simulink model "model_zad3"  (R2023a)
settings: Solver=ode45  StartTime=0.0  StopTime=600  RelTol=1e-3  EnableMultiTasking=on
values from neighbouring files (symbols this model uses):
  theta = [Gd.den{1}(2:3) Gd.num{1}(2:3)]'    [inicijalizacija.m]
  theta2 = [Gd2.den{1}(2:3) Gd2.num{1}(2:3)]'    [inicijalizacija.m]
  Ts = dt    [inicijalizacija.m]
libraries: simulink x2
settings Model: Creator=starcic  LastModifiedBy=Enio
settings SolverCC: AlgebraicLoopSolver=TrustRegion
settings DataIOCC: LimitDataPoints=on  SaveFormat=Array  ReturnWorkspaceOutputs=off
settings OptimizationCC: LifeSpan=inf
settings DebuggingCC: UnderspecifiedInitializationDetection=Classic  MergeDetectMultiDrivingBlocksExec=none  SolverPrmCheckMsg=warning  FcnCallInpInsideContextMsg=warning  UnconnectedInputMsg=warning  UnconnectedOutputMsg=warning  UnconnectedLineMsg=warning  StateNameClashWarn=warning  SFUnexpectedBacktrackingDiag=warning  SFNoUnconditionalDefaultTransitionDiag=warning  SFExecutionAtInitializationDiag=none  ArithmeticOperatorsInVariantConditions=warning
settings HardwareCC: ProdBitPerPointer=32  ProdBitPerSizeT=32  ProdBitPerPtrDiffT=32  ProdLargestAtomicFloat=None  ProdIntDivRoundTo=Undefined  ProdEndianess=Unspecified  ProdWordSize=32  ProdHWDeviceType=32-bit Generic
settings ModelReferenceCC: PropagateSignalLabelsOutOfModel=off
settings SFSimCC: SimUseLocalCustomCode=off  CustomCodeUndefinedFunction=UseInterfaceOnly
settings RTWCC: RTWUseLocalCustomCode=off
settings CodeAppCC: StateflowObjectComments=on
settings GRTTargetCC: TargetLangStandard=C89/C90 (ANSI)  CombineOutputUpdateFcns=off  GRTInterface=on
settings ConfigComp: CovMetricSettings=dw  CovSaveCumulativeToWorkspaceVar=on  CovSaveSingleToWorkspaceVar=on  CovExternalEMLEnable=off

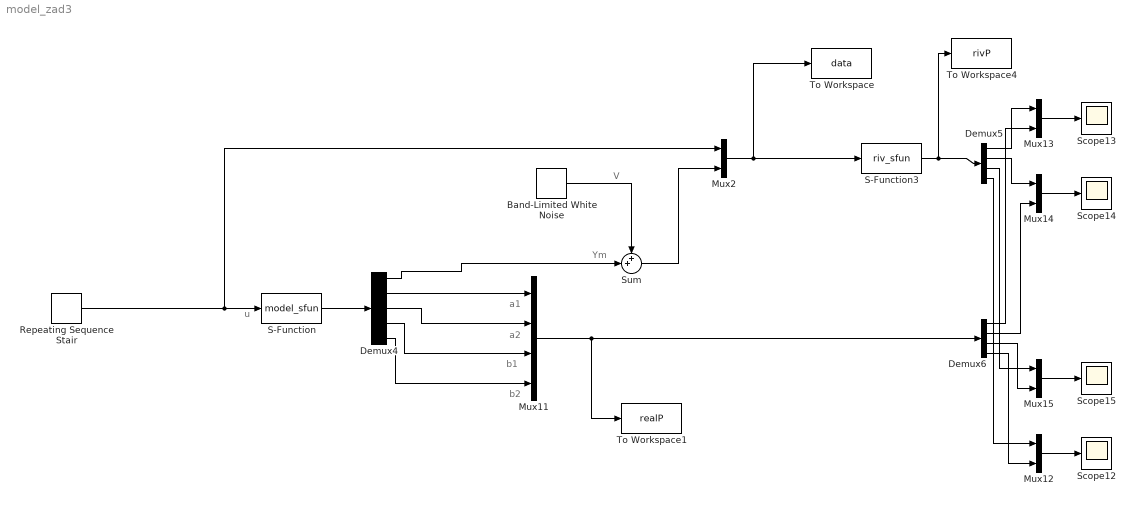
== system model_zad3 ==
  note: V
  note: u
  note: Ym
  note: b2
  note: b1
  note: a2
  note: a1
  Band-Limited White Noise : simulink/Sources/Band-Limited White Noise  Cov=[0.0000001]  Ts=Ts  seed=145656456
  Demux4 : Demux  Outputs=5
  Demux5 : Demux
  Demux6 : Demux
  Mux11 : Mux
  Mux{2,12..15} (5 alike) : Mux  Inputs=2
  Repeating Sequence Stair : simulink/Sources/Repeating Sequence Stair  OutValues=ui  tsamp=Ts  OutMin=[]  OutMax=[]  OutDataTypeStr=double  OutputDataTypeScalingMode=double  OutDataType=fixdt(0,8)  ConRadixGroup=Best Precision: Vector-wise  OutScaling=2^-12
  S-Function : S-Function  FunctionName=model_sfun  Parameters=theta,theta2  SFunctionDeploymentMode=off  EnableBusSupport=off
  S-Function3 : S-Function  FunctionName=riv_sfun  Parameters=Ts  SFunctionDeploymentMode=off  EnableBusSupport=off
  Scope{12..15} (4 alike) : Scope
  Sum : Sum  Inputs=++|
  To Workspace : ToWorkspace  VariableName=data  SaveFormat=Structure With Time  SampleTime=Ts
  To Workspace1 : ToWorkspace  VariableName=realP  SaveFormat=Structure With Time  SampleTime=Ts
  To Workspace4 : ToWorkspace  VariableName=rivP  SaveFormat=Structure With Time  SampleTime=Ts
  wires:
  Repeating Sequence Stair/1 -> Mux2/1, S-Function/1
  Mux2/1 -> S-Function3/1, To Workspace/1
  Sum/1 -> Mux2/2
  S-Function/1 -> Demux4/1
  Demux4/1 -> Sum/2
  Demux4/2 -> Mux11/1
  Demux4/3 -> Mux11/2
  Demux4/4 -> Mux11/3
  Demux4/5 -> Mux11/4
  S-Function3/1 -> To Workspace4/1, Demux5/1
  Mux11/1 -> To Workspace1/1, Demux6/1
  Demux5/1 -> Mux13/1
  Demux5/2 -> Mux14/1
  Demux5/3 -> Mux15/1
  Demux5/4 -> Mux12/1
  Demux6/1 -> Mux13/2
  Demux6/2 -> Mux14/2
  Demux6/3 -> Mux15/2
  Demux6/4 -> Mux12/2
  Mux13/1 -> Scope13/1
  Mux14/1 -> Scope14/1
  Mux15/1 -> Scope15/1
  Mux12/1 -> Scope12/1
  Band-Limited White Noise/1 -> Sum/1
